simulink model "Mesure_RoueGauche_BoucleOuverte"  (R2015a)
settings: Solver=FixedStepDiscrete  StartTime=0.0  StopTime=10  FixedStep=0.01  RelTol=1e-3
libraries: Wheels x1
settings Model: SimulationMode=external  ExtModeTrigDuration=2  Creator=tbaroche  LastModifiedBy=tbaroche
settings DataIOCC: MaxDataPoints=10000
settings OptimizationCC: OptimizeModelRefInitCode=on  LifeSpan=1
settings DebuggingCC: UnderspecifiedInitializationDetection=Classic  MergeDetectMultiDrivingBlocksExec=none
settings HardwareCC: ProdLargestAtomicInteger=Long  ProdLargestAtomicFloat=Double  ProdEndianess=LittleEndian  ProdHWDeviceType=ARM Compatible->ARM Cortex
settings RTWCC: SystemTargetFile=realtime.tlc  GenerateMakefile=off  TemplateMakefile=realtime.tmf  Description=Run on Target Hardware  RTWVerbose=off
settings ERTTargetCC: CombineOutputUpdateFcns=off  ExtModeTransport=3  ExtModeMexFile=ext_serial_win32_comm_rtt  ExtModeMexArgs=0 1 9600  ERTSrcFileBannerTemplate=realtime_code_template.cgt  ERTHdrFileBannerTemplate=realtime_code_template.cgt  ERTDataSrcFileTemplate=realtime_code_template.cgt  ERTDataHdrFileTemplate=realtime_code_template.cgt  ERTCustomFileTemplate=realtime_file_process.tlc

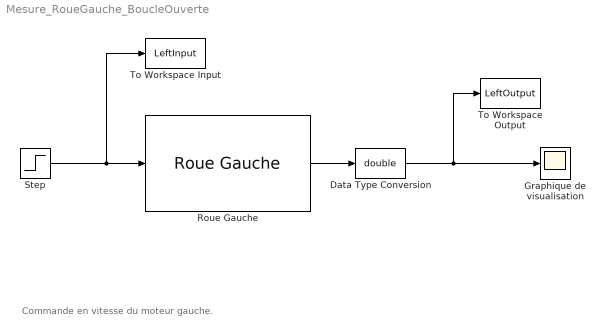
== system Mesure_RoueGauche_BoucleOuverte ==
  note: Commande en vitesse du moteur gauche.
  Data Type Conversion : DataTypeConversion  OutDataTypeStr=double
  Graphique de visualisation : Scope
  Roue Gauche : Wheels/Roue Gauche
  Step : Step  Time=3  After=50  SampleTime=0
  To Workspace Input : ToWorkspace  VariableName=LeftInput  SaveFormat=Structure With Time  SampleTime=-1
  To Workspace Output : ToWorkspace  VariableName=LeftOutput  SaveFormat=Structure With Time  SampleTime=-1
  wires:
  Roue Gauche/1 -> Data Type Conversion/1
  Step/1 -> Roue Gauche/1, To Workspace Input/1
  Data Type Conversion/1 -> To Workspace Output/1, Graphique de visualisation/1
